simulink model "Copy_of_analysis_discrete_hinf_ctrl_lin_model_z"  (R2020b)
settings: Solver=FixedStepAuto  StartTime=0.0  StopTime=10.0  FixedStep=1e-3  RelTol=1e-3
values from neighbouring files (symbols this model uses):
  B = 10    [hinfCostFunc.m]    (also in hinf_analysis_z.m; hinf_cmd_lmi.m = [zeros(4,2); Sigma.B]; init_rob_synth_sim.m; muCostFunc.m = 11)
  den_dis_hinf = tmp.Denominator{:}    [hinf_analysis_z.m]    (also in mu_analysis_z.m)
  dq0 = [0;0;0]    [hinfCostFunc.m]    (also in hinf_analysis_z.m; init_rob_synth_sim.m = [0; 0; 0]; muCostFunc.m; mu_analysis_z.m)
  K = 150    [hinfCostFunc.m]    (also in hinf_analysis_z.m; init_rob_synth_sim.m; muCostFunc.m = ureal('K',160,'Percentage',50); mu_analysis_z.m = ureal('K',160,'Percentage',50))
  M = 0.45    [hinfCostFunc.m]    (also in hinf_analysis_z.m; init_rob_synth_sim.m; muCostFunc.m = 0.42; mu_analysis_z.m = 0.42)
  num_dis_hinf = tmp.Numerator{:}    [hinf_analysis_z.m]    (also in mu_analysis_z.m)
  q0 = [1.676; -4.363; 1.497]    [hinfCostFunc.m]    (also in hinf_analysis_z.m; init_rob_synth_sim.m; muCostFunc.m; mu_analysis_z.m)
  Sigma = minreal(Sigma, [], false)    [hinfCostFunc.m]    (also in hinf_analysis_z.m = youbot_lin_model_ss_z; hinf_cmd_lmi.m = youbot_lin_model_ss_z; muCostFunc.m; mu_analysis_z.m = youbot_lin_model_ss_z)
  tau_m = 1/(10*2*pi)    (= 0.0159154943092)    [hinfCostFunc.m]    (also in hinf_analysis_z.m; init_rob_synth_sim.m; muCostFunc.m; mu_analysis_z.m)
settings Model: Creator=fortineau_vin  LastModifiedBy=Fortineau_Vin

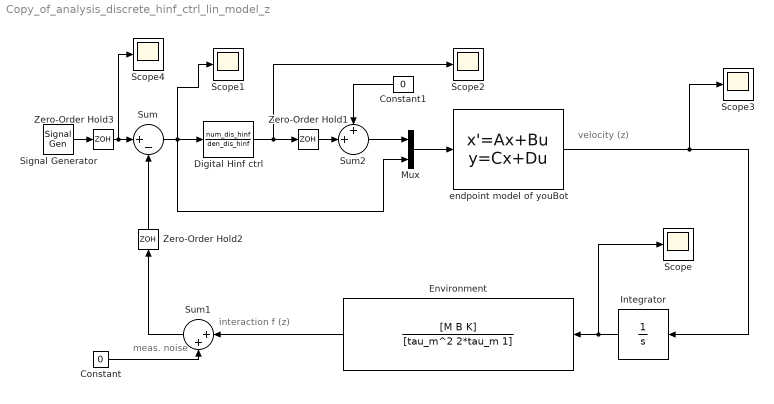
== system Copy_of_analysis_discrete_hinf_ctrl_lin_model_z ==
  note: interaction f (z)
  note: velocity (z)
  note: meas. noise
  Constant : Constant  Value=0
  Constant1 : Constant  Value=0
  Digital Hinf ctrl : TransferFcn  Numerator=num_dis_hinf  Denominator=den_dis_hinf
  Environment : TransferFcn  Numerator=[M B K]  Denominator=[tau_m^2 2*tau_m 1]
  Integrator : Integrator
  Mux : Mux  Inputs=2
  Scope{,1..4} (5 alike) : Scope
  Signal Generator : SignalGenerator  Frequency=2*pi  Units=rad/sec
  Sum : Sum  Inputs=|+-
  Sum1 : Sum  Inputs=|++
  Sum2 : Sum  Inputs=++|
  Zero-Order Hold1 : ZeroOrderHold  SampleTime=-1
  Zero-Order Hold2 : ZeroOrderHold  SampleTime=-1
  Zero-Order Hold3 : ZeroOrderHold  SampleTime=-1
  endpoint model of youBot : StateSpace  A=Sigma.A  B=Sigma.B  C=Sigma.C  D=Sigma.D  InitialCondition=[q0;dq0]
  wires:
  endpoint model of youBot/1 -> Scope3/1, Integrator/1
  Integrator/1 -> Scope/1, Environment/1
  Environment/1 -> Sum1/1
  Mux/1 -> endpoint model of youBot/1
  Sum/1 -> Scope1/1, Mux/2, Digital Hinf ctrl/1
  Sum1/1 -> Zero-Order Hold2/1
  Digital Hinf ctrl/1 -> Scope2/1, Zero-Order Hold1/1
  Sum2/1 -> Mux/1
  Constant1/1 -> Sum2/1
  Constant/1 -> Sum1/2
  Zero-Order Hold1/1 -> Sum2/2
  Zero-Order Hold2/1 -> Sum/2
  Signal Generator/1 -> Zero-Order Hold3/1
  Zero-Order Hold3/1 -> Scope4/1, Sum/1
